simulink model "pfc_desktop_hdl"  (R2024b)
settings: Solver=FixedStepDiscrete  StartTime=0.0  StopTime=.4  RelTol=1e-3
InitFcn:
  | fidelity_pfc_vals;
values from neighbouring files (symbols this model uses):
  fsw = 65    [fidelity_pfc_vals.m]
  Gs = 2e-2    (= 0.02)    [fidelity_pfc_vals.m]
  s = 1    [fidelity_pfc_vals.m]
  t_ss = tsw/30    (= 5.12820512821e-07)    [fidelity_pfc_vals.m]
  tsw = 1/(fsw*1e3)    (= 1.53846153846e-05)    [fidelity_pfc_vals.m]
undefined symbols (not defined in the file or in its folder): a, b, c, DiscIntNeverNeededParam
libraries: fl_lib x37, nesl_utility x31, hdlsllib x6, mcbcontrolslib x5, ee_lib x5, dspsrcs4 x3, slpidlib x2, simulink x1, spsSVPWMGenerator2LevelLib x1, spsPLL3phLib x1
(part 1 of 2)
settings Model: Creator=angro  LastModifiedBy=Angel
settings OptimizationCC: BlockReduction=off  ConditionallyExecuteInputs=off  DefaultParameterBehavior=Inlined
settings DebuggingCC: AlgebraicLoopMsg=error
settings HardwareCC: ProdBitPerPointer=32  ProdBitPerSizeT=32  ProdBitPerPtrDiffT=32  ProdLargestAtomicFloat=None  ProdIntDivRoundTo=Undefined  ProdEndianess=Unspecified  ProdWordSize=32  ProdHWDeviceType=ASIC/FPGA->ASIC/FPGA  TargetBitPerPointer=64  TargetBitPerSizeT=64  TargetBitPerPtrDiffT=64  TargetLongLongMode=on  TargetIntDivRoundTo=Zero  TargetEndianess=LittleEndian  TargetWordSize=64  TargetHWDeviceType=Custom Processor->MATLAB Host Computer  ProdEqTarget=off

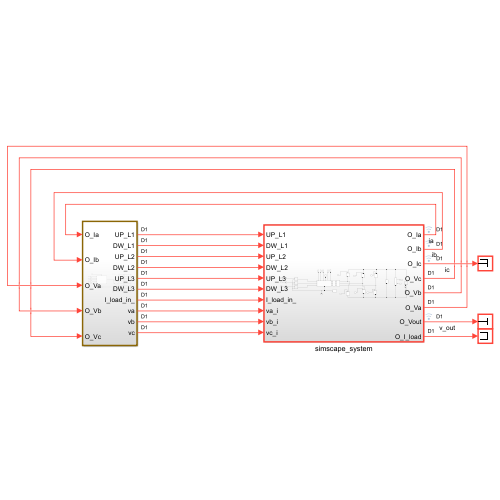
[thumbnail: Simulink's stored preview of the top-level diagram]
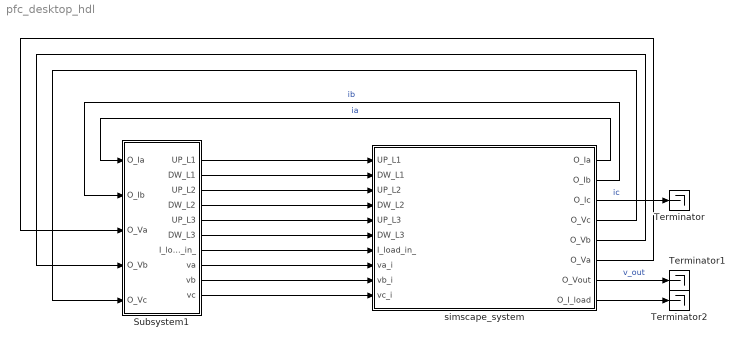
== system pfc_desktop_hdl ==
  Subsystem1 : Subsystem
  Terminator : Terminator
  Terminator1 : Terminator
  Terminator2 : Terminator
  simscape_system : Subsystem
  wires:
  simscape_system/1(O_Ia) -> Subsystem1/1(O_Ia)  "ia"
  simscape_system/6(O_Va) -> Subsystem1/3(O_Va)
  Subsystem1/5(UP_L3) -> simscape_system/5(UP_L3)
  Subsystem1/10(vc) -> simscape_system/10(vc_i)
  simscape_system/2(O_Ib) -> Subsystem1/2(O_Ib)  "ib"
  Subsystem1/9(vb) -> simscape_system/9(vb_i)
  Subsystem1/7(I_load_in_) -> simscape_system/7(I_load_in_)
  Subsystem1/3(UP_L2) -> simscape_system/3(UP_L2)
  Subsystem1/4(DW_L2) -> simscape_system/4(DW_L2)
  simscape_system/4(O_Vc) -> Subsystem1/5(O_Vc)
  Subsystem1/2(DW_L1) -> simscape_system/2(DW_L1)
  simscape_system/5(O_Vb) -> Subsystem1/4(O_Vb)
  simscape_system/3(O_Ic) -> Terminator/1  "ic"
  Subsystem1/6(DW_L3) -> simscape_system/6(DW_L3)
  simscape_system/8(O_I_load) -> Terminator2/1
  Subsystem1/1(UP_L1) -> simscape_system/1(UP_L1)
  simscape_system/7(O_Vout) -> Terminator1/1  "v_out"
  Subsystem1/8(va) -> simscape_system/8(va_i)

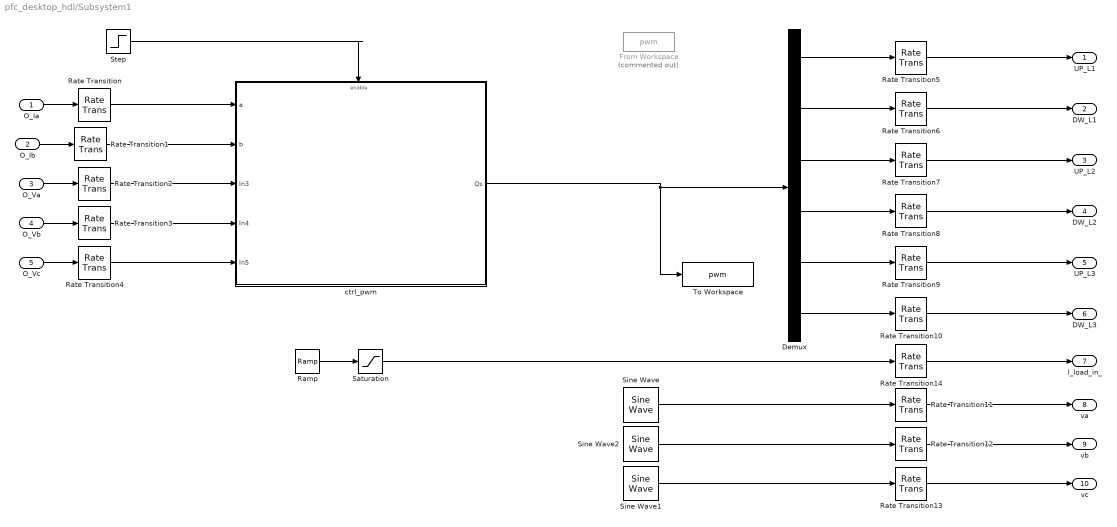
== system pfc_desktop_hdl/Subsystem1 ==
  O_Ia : Inport
  O_Ib : Inport  Port=2
  O_Va : Inport  Port=3
  O_Vb : Inport  Port=4
  O_Vc : Inport  Port=5
  Demux : Demux  Outputs=6
  From Workspace : FromWorkspace  Commented=on  VariableName=pwm  SampleTime=t_ss  Interpolate=off  ZeroCross=off  OutputAfterFinalValue=Holding final value
  Ramp : simulink/Sources/Ramp  slope=1/50  start=2/50  InitialOutput=0
  Rate Transition{,1..4,14} (6 alike) : RateTransition  OutPortSampleTime=t_ss
  Rate Transition{5..13} (9 alike) : RateTransition
  Saturation : Saturate  UpperLimit=2
  Sine Wave : dspsrcs4/Sine Wave  Amplitude=325  Frequency=50  Phase=0  SampleMode=Discrete  OutComplex=Real  CompMethod=Table lookup  TableSize=Speed  SampleTime=tsw  SamplesPerFrame=1  ResetState=Restart at time zero  OutputFrames=off  dataType=double  wordLen=16  udDataType=sfix(16)  fracBitsMode=Best precision  numFracBits=15  OutDataTypeStr=double  LastOutDataTypeStr=double
  Sine Wave1 : dspsrcs4/Sine Wave  Amplitude=325  Frequency=50  Phase=2*pi/3  SampleMode=Discrete  OutComplex=Real  CompMethod=Table lookup  TableSize=Speed  SampleTime=tsw  SamplesPerFrame=1  ResetState=Restart at time zero  OutputFrames=off  dataType=double  wordLen=16  udDataType=sfix(16)  fracBitsMode=Best precision  numFracBits=15  OutDataTypeStr=double  LastOutDataTypeStr=double
  Sine Wave2 : dspsrcs4/Sine Wave  Amplitude=325  Frequency=50  Phase=-2*pi/3  SampleMode=Discrete  OutComplex=Real  CompMethod=Table lookup  TableSize=Speed  SampleTime=tsw  SamplesPerFrame=1  ResetState=Restart at time zero  OutputFrames=off  dataType=double  wordLen=16  udDataType=sfix(16)  fracBitsMode=Best precision  numFracBits=15  OutDataTypeStr=double  LastOutDataTypeStr=double
  Step : Step  Time=2/50  SampleTime=0
  To Workspace : ToWorkspace  VariableName=pwm  SaveFormat=Timeseries  SampleTime=-1
  ctrl_pwm : Subsystem
  UP_L1 : Outport
  DW_L1 : Outport  Port=2
  UP_L2 : Outport  Port=3
  DW_L2 : Outport  Port=4
  UP_L3 : Outport  Port=5
  DW_L3 : Outport  Port=6
  I_load_in_ : Outport  Port=7
  va : Outport  Port=8
  vb : Outport  Port=9
  vc : Outport  Port=10
  wires:
  Demux/5 -> Rate Transition9/1
  Demux/1 -> Rate Transition5/1
  Demux/6 -> Rate Transition10/1
  Demux/4 -> Rate Transition8/1
  Demux/3 -> Rate Transition7/1
  Demux/2 -> Rate Transition6/1
  O_Ia/1 -> Rate Transition/1
  O_Ib/1 -> Rate Transition1/1
  O_Va/1 -> Rate Transition2/1
  O_Vb/1 -> Rate Transition3/1
  O_Vc/1 -> Rate Transition4/1
  Rate Transition5/1 -> UP_L1/1
  Rate Transition6/1 -> DW_L1/1
  Rate Transition7/1 -> UP_L2/1
  Rate Transition8/1 -> DW_L2/1
  Rate Transition9/1 -> UP_L3/1
  Rate Transition10/1 -> DW_L3/1
  Saturation/1 -> Rate Transition14/1
  Sine Wave/1 -> Rate Transition11/1
  Sine Wave2/1 -> Rate Transition12/1
  Sine Wave1/1 -> Rate Transition13/1
  Rate Transition11/1 -> va/1
  Rate Transition12/1 -> vb/1
  Rate Transition13/1 -> vc/1
  ctrl_pwm/1(Qs) -> Demux/1, To Workspace/1
  Rate Transition/1 -> ctrl_pwm/1(a)
  Rate Transition1/1 -> ctrl_pwm/2(b)
  Rate Transition2/1 -> ctrl_pwm/3(In3)
  Rate Transition3/1 -> ctrl_pwm/4(In4)
  Rate Transition4/1 -> ctrl_pwm/5(In5)
  Step/1 -> ctrl_pwm/Enable
  Rate Transition14/1 -> I_load_in_/1
  Ramp/1 -> Saturation/1

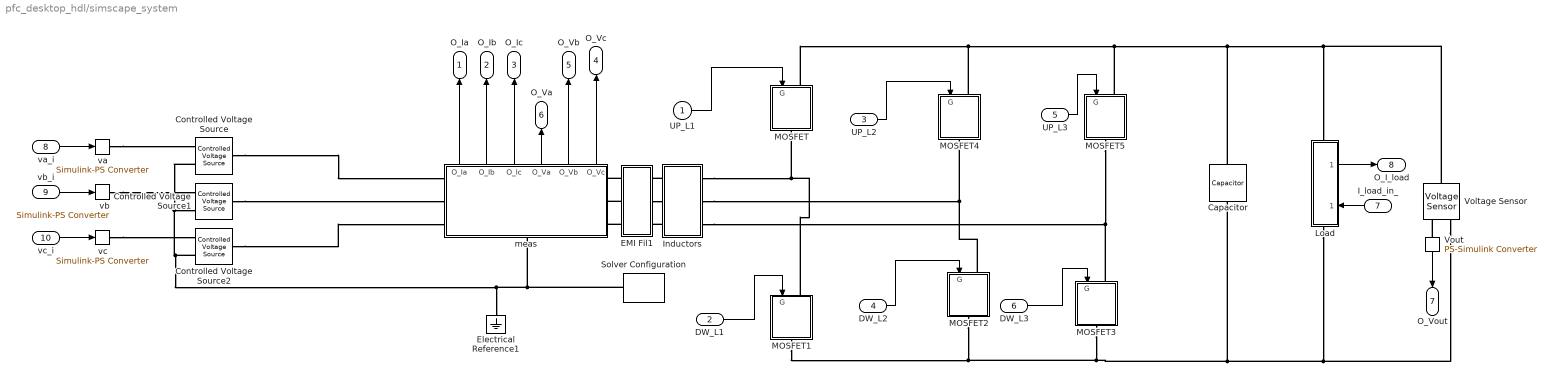
== system pfc_desktop_hdl/simscape_system ==
  UP_L1 : Inport
  DW_L1 : Inport  Port=2
  UP_L2 : Inport  Port=3
  DW_L2 : Inport  Port=4
  UP_L3 : Inport  Port=5
  DW_L3 : Inport  Port=6
  I_load_in_ : Inport  Port=7
  va_i : Inport  Port=8
  vb_i : Inport  Port=9
  vc_i : Inport  Port=10
  Capacitor : ee_lib/Passive/Capacitor  cap_option=ee.enum.passive.capacitor.capOption.const  c=c_out uF  Cvec=[1e-05, 1e-06] F  Vvec=[0, 10] V  CV_table_symmetry=1  f_vec=[1, 10] kHz  DFext_vec=[.8, 1.2]  enable_C_tol=0  averaging_period=0 s  C_tol=5  tol_distribution=1  nSigma=4  r=1e-3*6 Ohm  g=0 1/Ohm  enable_operating_limits=0  operating_limit_action=2  max_working_voltage_range=[-25, 25] V  power_rating=1 W  maxTemperature=85 degC  thermalEnable=false  thermalMass=1 J/K  fault_action=simscape.enum.assert.action.none  t_fault=1 s  i_specify=off  i_priority=None  i=0 A  i_nominal_specify=off  i_nominal_value=1  i_nominal_unit=A  v_specify=off  v_priority=None  v=0 V  v_nominal_specify=off  v_nominal_value=1  v_nominal_unit=V  vc_specify=on  vc_priority=High  vc=580 V  vc_nominal_specify=off  vc_nominal_value=1  vc_nominal_unit=V  T_specify=off  T_priority=None  T=298.15 K  T_nominal_specify=off  T_nominal_value=1  T_nominal_unit=K
  Controlled Voltage Source : fl_lib/Electrical/Electrical Sources/Controlled Voltage Source
  Controlled Voltage Source1 : fl_lib/Electrical/Electrical Sources/Controlled Voltage Source
  Controlled Voltage Source2 : fl_lib/Electrical/Electrical Sources/Controlled Voltage Source
  EMI Fil1 : Subsystem
  Electrical Reference1 : fl_lib/Electrical/Electrical Elements/Electrical Reference
  Inductors : Subsystem
  Load : Subsystem
      settings: PortSchema="{\"entries\":[{\"content\":{\"sides\":[{\"content\":{\"connectorIds\":[\"LConn1\"]},\"type\":\"ConnectorPlacement.EquallySpacedRectSide\",\"uuid\":\"effb2338-687f-46f5-a36d-064d1cdd1f89\"},{\"content\":{\"connectorIds\":[\"RConn1\"],\"side\":\"RIGHT\"},\"type\":\"ConnectorPlacement.EquallySpacedRectSide\",\"uuid\":\"901d8297-0f3f-4280-ade7-978b42e696ee\"},{\"content\":{\"side\":\"TOP\"},\"type\":\"ConnectorPlacement.EquallySpacedRectSide\",\"uuid\":\"94ece1e5-b3d1-4ff8-a800-be801e6d950f\"},{\"content\":{\"connectorIds\":[\"In1\",\"Out1\"],\"side\":\"BOTTOM\"},\"type\":\"ConnectorPlacement.EquallySpacedRectSide\",\"uuid\":\"36082d89-7906-4f78-be00-891e05fea0eb\"}]},\"type\":\"ConnectorPlacement.EquallySpacedConnector\",\"uuid\":\"9e7f386b-2a06-43cf-bdf5-65e67bd802eb\"}],\"packageUris\":[\"http://schema.mathworks.com/mf0/Connector/R2020b\"],\"version\":\"1.0\"}"
  MOSFET : Subsystem
      settings: CopyFcn=set_param(gcb, 'LinkStatus', 'none');
  MOSFET1 : Subsystem
      settings: CopyFcn=set_param(gcb, 'LinkStatus', 'none');
  MOSFET2 : Subsystem
      settings: CopyFcn=set_param(gcb, 'LinkStatus', 'none');
  MOSFET3 : Subsystem
      settings: CopyFcn=set_param(gcb, 'LinkStatus', 'none');
  MOSFET4 : Subsystem
      settings: CopyFcn=set_param(gcb, 'LinkStatus', 'none');
  MOSFET5 : Subsystem
      settings: CopyFcn=set_param(gcb, 'LinkStatus', 'none');
  Solver Configuration : nesl_utility/Solver Configuration  PhysicalDomain=network_engine_domain  SubClassName=solver  LeftPortType=input  RightPortType=generic  Tones=[]  Harmonics=[]  SimulateNoise=off  Profile=off  UseLocalSampling=off  EnableSwitchedLinearOptims=on  FrequencyDomain=off  UseCCode=off  RelTol=0.001  AbsTol=1e-06  MinStep=1e-09  ToWorkspace=off  RevertToSquareIcSolve=off  NumHomotopyIterations=100  PhasorMode=off  PhasorModeNumHarmonics=1  ConsistencySolver=NEWTON_FTOL  IndexReductionMethod=None  DoDC=off  ResidualTolerance=1e-6  ConsistencyTolSource=GLOBAL  ConsistencyAbsTol=0.001  ConsistencyRelTol=0.001  ConsistencyTolFactor=0.001  UseLocalSolver=on  LocalSolverChoice=NE_BACKWARD_EULER_ADVANCER  ResolveIndetEquations=on  FunctionEvalNumThread=1  LocalSolverSampleTime=t_ss  DoFixedCost=on  MaxNonlinIter=1  MaxModeIter=10  ComputeImpulses=off  ImpulseIterations=2  LinearAlgebra=auto  LinearAlgebraNumThread=0  EquationFormulation=NE_TIME_EF  DelaysMemoryBudget=1024  AutomaticFiltering=off  FilteringTimeConstant=0.001  PartitionStorageMethod=EXHAUSTIVE  PartitionMemoryBudget=1024  PartitionMethod=ROBUST  MultibodyUseLocalSolver=off  MultibodyLocalSolverChoice=ODE1  MultibodyLocalSolverSampleTime=0.001
  Voltage Sensor : fl_lib/Electrical/Electrical Sensors/Voltage Sensor
  Vout : nesl_utility/PS-Simulink Converter  PhysicalDomain=network_engine_domain  SubClassName=ps_output  LeftPortType=input  RightPortType=output  PseudoPeriodic=off  Frequencies=[]  VectorFormat=1-D array  Unit=V  AffineConversion=off
  meas : Subsystem
      settings: PortSchema="{\"entries\":[{\"content\":{\"sides\":[{\"content\":{\"connectorIds\":[\"LConn1\",\"LConn2\",\"LConn3\"]},\"type\":\"ConnectorPlacement.EquallySpacedRectSide\",\"uuid\":\"63fb0446-2195-41ce-9f27-949cb83cb3c9\"},{\"content\":{\"connectorIds\":[\"RConn1\",\"RConn2\",\"RConn3\"],\"side\":\"RIGHT\"},\"type\":\"ConnectorPlacement.EquallySpacedRectSide\",\"uuid\":\"9968c418-1dbf-4d06-ba5c-e609e6b84d90\"},{\"content\":{\"connectorIds\":[\"Out1\",\"Out2\",\"Out3\",\"Out4\",\"Out5\",\"Out6\"],\"side\":\"TOP\"},\"type\":\"ConnectorPlacement.EquallySpacedRectSide\",\"uuid\":\"bf7c2fdb-620d-435f-9b2a-06b2c14c987c\"},{\"content\":{\"connectorIds\":[\"RConn4\"],\"side\":\"BOTTOM\"},\"type\":\"ConnectorPlacement.EquallySpacedRectSide\",\"uuid\":\"eb9cce3f-153e-47a2-a171-a4890e03f4a1\"}]},\"type\":\"ConnectorPlacement.EquallySpacedConnector\",\"uuid\":\"4b9ac32f-b167-4dce-a874-653844c6cf4c\"}],\"packageUris\":[\"http://schema.mathworks.com/mf0/Connector/R2020b\"],\"version\":\"1.0\"}"
  va : nesl_utility/Simulink-PS Converter  PhysicalDomain=network_engine_domain  SubClassName=ps_input  LeftPortType=input  RightPortType=output  PseudoPeriodic=off  Frequencies=[]  NoiseDistribution=none  NoiseParameters=[]  Unit=V  AffineConversion=off  FilteringAndDerivatives=zero  SimscapeFilterOrder=1  InputFilterTimeConstant=0.001  UdotUserProvided=0
  vb : nesl_utility/Simulink-PS Converter  PhysicalDomain=network_engine_domain  SubClassName=ps_input  LeftPortType=input  RightPortType=output  PseudoPeriodic=off  Frequencies=[]  NoiseDistribution=none  NoiseParameters=[]  Unit=V  AffineConversion=off  FilteringAndDerivatives=zero  SimscapeFilterOrder=1  InputFilterTimeConstant=0.001  UdotUserProvided=0
  vc : nesl_utility/Simulink-PS Converter  PhysicalDomain=network_engine_domain  SubClassName=ps_input  LeftPortType=input  RightPortType=output  PseudoPeriodic=off  Frequencies=[]  NoiseDistribution=none  NoiseParameters=[]  Unit=V  AffineConversion=off  FilteringAndDerivatives=zero  SimscapeFilterOrder=1  InputFilterTimeConstant=0.001  UdotUserProvided=0
  O_Ia : Outport
  O_Ib : Outport  Port=2
  O_Ic : Outport  Port=3
  O_Vc : Outport  Port=4
  O_Vb : Outport  Port=5
  O_Va : Outport  Port=6
  O_Vout : Outport  Port=7
  O_I_load : Outport  Port=8
  wires:
  DW_L1/1 -> MOSFET1/1(G)
  UP_L3/1 -> MOSFET5/1(G)
  UP_L2/1 -> MOSFET4/1(G)
  DW_L3/1 -> MOSFET3/1(G)
  UP_L1/1 -> MOSFET/1(G)
  DW_L2/1 -> MOSFET2/1(G)
  Vout/1 -> O_Vout/1
  I_load_in_/1 -> Load/1(I_load_in_)
  meas/1(O_Ia) -> O_Ia/1
  meas/2(O_Ib) -> O_Ib/1
  meas/3(O_Ic) -> O_Ic/1
  meas/6(O_Vc) -> O_Vc/1
  meas/5(O_Vb) -> O_Vb/1
  meas/4(O_Va) -> O_Va/1
  va_i/1 -> va/1
  vb_i/1 -> vb/1
  vc_i/1 -> vc/1
  Load/1(O_I_load) -> O_I_load/1
  connections:
  Controlled Voltage Source/RConn2 -- Electrical Reference1/LConn1 -- Solver Configuration/RConn1 -- meas/RConn4 -- Controlled Voltage Source2/RConn2 -- Controlled Voltage Source1/RConn2
  Inductors/LConn1 -- EMI Fil1/RConn1
  EMI Fil1/RConn2 -- Inductors/LConn2
  Inductors/LConn3 -- EMI Fil1/RConn3
  Capacitor/LConn1 -- MOSFET5/LConn1 -- MOSFET4/LConn1 -- MOSFET/LConn1 -- Voltage Sensor/LConn1 -- Load/RConn1
  va/RConn1 -- Controlled Voltage Source/RConn1
  vb/RConn1 -- Controlled Voltage Source1/RConn1
  vc/RConn1 -- Controlled Voltage Source2/RConn1
  Controlled Voltage Source/LConn1 -- meas/LConn1
  Controlled Voltage Source1/LConn1 -- meas/LConn2
  Controlled Voltage Source2/LConn1 -- meas/LConn3
  EMI Fil1/LConn1 -- meas/RConn1
  EMI Fil1/LConn2 -- meas/RConn2
  EMI Fil1/LConn3 -- meas/RConn3
  Inductors/RConn1 -- MOSFET1/LConn1 -- MOSFET/RConn1
  Inductors/RConn2 -- MOSFET4/RConn1 -- MOSFET2/LConn1
  Inductors/RConn3 -- MOSFET5/RConn1 -- MOSFET3/LConn1
  Load/LConn1 -- Voltage Sensor/RConn2 -- MOSFET3/RConn1 -- MOSFET2/RConn1 -- MOSFET1/RConn1 -- Capacitor/RConn1
  Vout/LConn1 -- Voltage Sensor/RConn1

== system pfc_desktop_hdl/Subsystem1/ctrl_pwm ==
  a : Inport
  b : Inport  Port=2
  In3 : Inport  Port=3
  In4 : Inport  Port=4
  In5 : Inport  Port=5
  Enable : EnablePort
  PI_CTRL : Subsystem
  SVPWM : Subsystem
  transforms : Subsystem
  Qs : Outport
  wires:
  transforms/1(id) -> PI_CTRL/1(id)
  transforms/3(angle) -> SVPWM/2(angle)
  PI_CTRL/1(Vd_inductor) -> SVPWM/1(Vd_inductor)
  a/1 -> transforms/1(a)
  In5/1 -> transforms/5(In5)
  transforms/2(iq) -> PI_CTRL/2(iq)
  SVPWM/1(P) -> Qs/1  "Qs"
  PI_CTRL/2(Vq_inductor) -> SVPWM/3(Vq_inductor)
  b/1 -> transforms/2(b)
  In3/1 -> transforms/3(In3)
  In4/1 -> transforms/4(In4)

== system pfc_desktop_hdl/simscape_system/EMI Fil1 ==
  Coupled Lines (Three-Phase) : ee_lib/Passive/Lines/Coupled Lines (Three-Phase)  prm=1  La=1e-3 H  Lb=1e-3 H  Lc=1e-3 H  L=10 mH  Lmab=3e-4 H  Lmac=3e-4 H  Lmbc=3e-4 H  Lm=0 mH  Ra=0.001 Ohm  Rb=0.001 Ohm  Rc=0.001 Ohm  R=0.001 Ohm  Rm=0 Ohm  Ga=1e-9 1/Ohm  Gb=1e-9 1/Ohm  Gc=1e-9 1/Ohm  G=1e-9 1/Ohm  I_L_specify=off  I_L_priority=High  I_L=[0, 0, 0] A  I_L_nominal_specify=off  I_L_nominal_value=1  I_L_nominal_unit=A  i_La_specify=off  i_La_priority=High  i_La=0 A  i_La_nominal_specify=off  i_La_nominal_value=1  i_La_nominal_unit=A  i_Lb_specify=off  i_Lb_priority=High  i_Lb=0 A  i_Lb_nominal_specify=off  i_Lb_nominal_value=1  i_Lb_nominal_unit=A  i_Lc_specify=off  i_Lc_priority=High  i_Lc=0 A  i_Lc_nominal_specify=off  i_Lc_nominal_value=1  i_Lc_nominal_unit=A
      settings: InternalSimscapePortConfiguration="{\"Bottom\":[],\"Left\":[{\"id\":\"a1\",\"label\":\"a1\",\"type\":\"foundation.electrical.electrical\"},{\"id\":\"b1\",\"label\":\"b1\",\"type\":\"foundation.electrical.electrical\"},{\"id\":\"c1\",\"label\":\"c1\",\"type\":\"foundation.electrical.electrical\"}],\"Right\":[{\"id\":\"a2\",\"label\":\"a2\",\"type\":\"foundation.electrical.electrical\"},{\"id\":\"b2\",\"label\":\"b2\",\"type\":\"foundation.electrical.electrical\"},{\"id\":\"c2\",\"label\":\"c2\",\"type\":\"foundation.electrical.electrical\"}],\"Top\":[]}"
  +A : PMIOPort  Side=Left
  +B : PMIOPort  Port=2  Side=Left
  +C : PMIOPort  Port=3  Side=Left
  -A : PMIOPort  Port=4  Side=Right
  -B : PMIOPort  Port=5  Side=Right
  -C : PMIOPort  Port=6  Side=Right
  connections:
  Coupled Lines (Three-Phase)/LConn1 -- +A/RConn1
  +C/RConn1 -- Coupled Lines (Three-Phase)/LConn3
  -C/RConn1 -- Coupled Lines (Three-Phase)/RConn3
  -B/RConn1 -- Coupled Lines (Three-Phase)/RConn2
  +B/RConn1 -- Coupled Lines (Three-Phase)/LConn2
  -A/RConn1 -- Coupled Lines (Three-Phase)/RConn1

== system pfc_desktop_hdl/simscape_system/Inductors ==
  Inductor : ee_lib/Passive/Inductor  l=l_ind uH  enable_L_tol=0  L_tol=0  tol_distribution=1  nSigma=4  r=1e-3 Ohm  g=1e-9 1/Ohm  enable_operating_limits=0  operating_limit_action=2  max_working_current=1 A  power_rating=1 W  fault_action=simscape.enum.assert.action.none  t_fault=1 s  i_L_specify=off  i_L_priority=High  i_L=0 A  i_L_nominal_specify=off  i_L_nominal_value=1  i_L_nominal_unit=A
  Inductor1 : ee_lib/Passive/Inductor  l=l_ind uH  enable_L_tol=0  L_tol=0  tol_distribution=1  nSigma=4  r=1e-3 Ohm  g=1e-9 1/Ohm  enable_operating_limits=0  operating_limit_action=2  max_working_current=1 A  power_rating=1 W  fault_action=simscape.enum.assert.action.none  t_fault=1 s  i_L_specify=off  i_L_priority=High  i_L=0 A  i_L_nominal_specify=off  i_L_nominal_value=1  i_L_nominal_unit=A
  Inductor2 : ee_lib/Passive/Inductor  l=l_ind uH  enable_L_tol=0  L_tol=0  tol_distribution=1  nSigma=4  r=1e-3 Ohm  g=1e-9 1/Ohm  enable_operating_limits=0  operating_limit_action=2  max_working_current=1 A  power_rating=1 W  fault_action=simscape.enum.assert.action.none  t_fault=1 s  i_L_specify=off  i_L_priority=High  i_L=0 A  i_L_nominal_specify=off  i_L_nominal_value=1  i_L_nominal_unit=A
  IAout : PMIOPort  Side=Right
  IA : PMIOPort  Port=2  Side=Left
  Ib : PMIOPort  Port=3  Side=Left
  IBout : PMIOPort  Port=4  Side=Right
  IC : PMIOPort  Port=5  Side=Left
  ICout : PMIOPort  Port=6  Side=Right
  connections:
  Ib/RConn1 -- Inductor/LConn1
  IBout/RConn1 -- Inductor/RConn1
  IAout/RConn1 -- Inductor2/RConn1
  Inductor2/LConn1 -- IA/RConn1
  Inductor1/LConn1 -- IC/RConn1
  ICout/RConn1 -- Inductor1/RConn1

== system pfc_desktop_hdl/simscape_system/Load ==
  I_load_in_ : Inport
  Controlled Current Source : fl_lib/Electrical/Electrical Sources/Controlled Current Source
  Current Sensor : fl_lib/Electrical/Electrical Sensors/Current Sensor
  I_load : nesl_utility/PS-Simulink Converter  PhysicalDomain=network_engine_domain  SubClassName=ps_output  LeftPortType=input  RightPortType=output  PseudoPeriodic=off  Frequencies=[]  VectorFormat=1-D array  Unit=inherit  AffineConversion=off
  I_load_in : nesl_utility/Simulink-PS Converter  PhysicalDomain=network_engine_domain  SubClassName=ps_input  LeftPortType=input  RightPortType=output  PseudoPeriodic=off  Frequencies=[]  NoiseDistribution=none  NoiseParameters=[]  Unit=1  AffineConversion=off  FilteringAndDerivatives=zero  SimscapeFilterOrder=1  InputFilterTimeConstant=0.001  UdotUserProvided=0
  Iout : PMIOPort  Side=Left
  Iin : PMIOPort  Port=2  Side=Right
  O_I_load : Outport
  wires:
  I_load_in_/1 -> I_load_in/1
  I_load/1 -> O_I_load/1
  connections:
  Current Sensor/LConn1 -- Controlled Current Source/LConn1
  Controlled Current Source/RConn2 -- Iin/RConn1
  I_load_in/RConn1 -- Controlled Current Source/RConn1
  I_load/LConn1 -- Current Sensor/RConn1
  Current Sensor/RConn2 -- Iout/RConn1

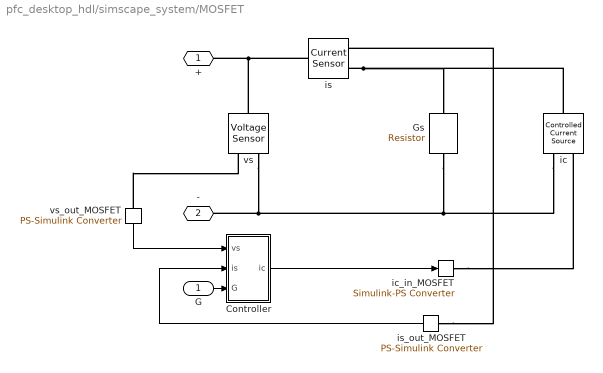
== system pfc_desktop_hdl/simscape_system/MOSFET ==
  G : Inport
  Controller : Subsystem
  Gs : fl_lib/Electrical/Electrical Elements/Resistor  R=1/Gs Ohm  i_specify=off  i_priority=None  i=0 A  i_nominal_specify=off  i_nominal_value=1  i_nominal_unit=A  v_specify=off  v_priority=None  v=0 V  v_nominal_specify=off  v_nominal_value=1  v_nominal_unit=V
  ic : fl_lib/Electrical/Electrical Sources/Controlled Current Source
  ic_in_MOSFET : nesl_utility/Simulink-PS Converter  PhysicalDomain=network_engine_domain  SubClassName=ps_input  LeftPortType=input  RightPortType=output  PseudoPeriodic=off  Frequencies=[]  NoiseDistribution=none  NoiseParameters=[]  Unit=A  AffineConversion=off  FilteringAndDerivatives=provide  SimscapeFilterOrder=1  InputFilterTimeConstant=0.001  UdotUserProvided=0
  is : fl_lib/Electrical/Electrical Sensors/Current Sensor
  is_out_MOSFET : nesl_utility/PS-Simulink Converter  PhysicalDomain=network_engine_domain  SubClassName=ps_output  LeftPortType=input  RightPortType=output  PseudoPeriodic=off  Frequencies=[]  VectorFormat=1-D array  Unit=A  AffineConversion=off
  vs : fl_lib/Electrical/Electrical Sensors/Voltage Sensor
  vs_out_MOSFET : nesl_utility/PS-Simulink Converter  PhysicalDomain=network_engine_domain  SubClassName=ps_output  LeftPortType=input  RightPortType=output  PseudoPeriodic=off  Frequencies=[]  VectorFormat=1-D array  Unit=V  AffineConversion=off
  + : PMIOPort  Side=Left
  - : PMIOPort  Port=2  Side=Right
  wires:
  Controller/1(ic) -> ic_in_MOSFET/1
  G/1 -> Controller/3(G)
  is_out_MOSFET/1 -> Controller/2(is)
  vs_out_MOSFET/1 -> Controller/1(vs)
  connections:
  is_out_MOSFET/LConn1 -- is/RConn1
  vs_out_MOSFET/LConn1 -- vs/RConn1
  ic_in_MOSFET/RConn1 -- ic/RConn1
  is/LConn1 -- +/RConn1 -- vs/LConn1
  ic/RConn2 -- Gs/RConn1 -- -/RConn1 -- vs/RConn2
  is/RConn2 -- Gs/LConn1 -- ic/LConn1

== system pfc_desktop_hdl/simscape_system/MOSFET1 ==
  G : Inport
  Controller : Subsystem
  Gs : fl_lib/Electrical/Electrical Elements/Resistor  R=1/Gs Ohm  i_specify=off  i_priority=None  i=0 A  i_nominal_specify=off  i_nominal_value=1  i_nominal_unit=A  v_specify=off  v_priority=None  v=0 V  v_nominal_specify=off  v_nominal_value=1  v_nominal_unit=V
  ic : fl_lib/Electrical/Electrical Sources/Controlled Current Source
  ic_in_MOSFET : nesl_utility/Simulink-PS Converter  PhysicalDomain=network_engine_domain  SubClassName=ps_input  LeftPortType=input  RightPortType=output  PseudoPeriodic=off  Frequencies=[]  NoiseDistribution=none  NoiseParameters=[]  Unit=A  AffineConversion=off  FilteringAndDerivatives=provide  SimscapeFilterOrder=1  InputFilterTimeConstant=0.001  UdotUserProvided=0
  is : fl_lib/Electrical/Electrical Sensors/Current Sensor
  is_out_MOSFET : nesl_utility/PS-Simulink Converter  PhysicalDomain=network_engine_domain  SubClassName=ps_output  LeftPortType=input  RightPortType=output  PseudoPeriodic=off  Frequencies=[]  VectorFormat=1-D array  Unit=A  AffineConversion=off
  vs : fl_lib/Electrical/Electrical Sensors/Voltage Sensor
  vs_out_MOSFET : nesl_utility/PS-Simulink Converter  PhysicalDomain=network_engine_domain  SubClassName=ps_output  LeftPortType=input  RightPortType=output  PseudoPeriodic=off  Frequencies=[]  VectorFormat=1-D array  Unit=V  AffineConversion=off
  + : PMIOPort  Side=Left
  - : PMIOPort  Port=2  Side=Right
  wires:
  vs_out_MOSFET/1 -> Controller/1(vs)
  is_out_MOSFET/1 -> Controller/2(is)
  G/1 -> Controller/3(G)
  Controller/1(ic) -> ic_in_MOSFET/1
  connections:
  ic/LConn1 -- Gs/LConn1 -- is/RConn2
  vs/RConn2 -- -/RConn1 -- Gs/RConn1 -- ic/RConn2
  vs/LConn1 -- +/RConn1 -- is/LConn1
  ic_in_MOSFET/RConn1 -- ic/RConn1
  vs_out_MOSFET/LConn1 -- vs/RConn1
  is_out_MOSFET/LConn1 -- is/RConn1

== system pfc_desktop_hdl/simscape_system/MOSFET2 ==
  G : Inport
  Controller : Subsystem
  Gs : fl_lib/Electrical/Electrical Elements/Resistor  R=1/Gs Ohm  i_specify=off  i_priority=None  i=0 A  i_nominal_specify=off  i_nominal_value=1  i_nominal_unit=A  v_specify=off  v_priority=None  v=0 V  v_nominal_specify=off  v_nominal_value=1  v_nominal_unit=V
  ic : fl_lib/Electrical/Electrical Sources/Controlled Current Source
  ic_in_MOSFET : nesl_utility/Simulink-PS Converter  PhysicalDomain=network_engine_domain  SubClassName=ps_input  LeftPortType=input  RightPortType=output  PseudoPeriodic=off  Frequencies=[]  NoiseDistribution=none  NoiseParameters=[]  Unit=A  AffineConversion=off  FilteringAndDerivatives=provide  SimscapeFilterOrder=1  InputFilterTimeConstant=0.001  UdotUserProvided=0
  is : fl_lib/Electrical/Electrical Sensors/Current Sensor
  is_out_MOSFET : nesl_utility/PS-Simulink Converter  PhysicalDomain=network_engine_domain  SubClassName=ps_output  LeftPortType=input  RightPortType=output  PseudoPeriodic=off  Frequencies=[]  VectorFormat=1-D array  Unit=A  AffineConversion=off
  vs : fl_lib/Electrical/Electrical Sensors/Voltage Sensor
  vs_out_MOSFET : nesl_utility/PS-Simulink Converter  PhysicalDomain=network_engine_domain  SubClassName=ps_output  LeftPortType=input  RightPortType=output  PseudoPeriodic=off  Frequencies=[]  VectorFormat=1-D array  Unit=V  AffineConversion=off
  + : PMIOPort  Side=Left
  - : PMIOPort  Port=2  Side=Right
  wires:
  Controller/1(ic) -> ic_in_MOSFET/1
  G/1 -> Controller/3(G)
  is_out_MOSFET/1 -> Controller/2(is)
  vs_out_MOSFET/1 -> Controller/1(vs)
  connections:
  is_out_MOSFET/LConn1 -- is/RConn1
  vs_out_MOSFET/LConn1 -- vs/RConn1
  ic_in_MOSFET/RConn1 -- ic/RConn1
  is/LConn1 -- +/RConn1 -- vs/LConn1
  ic/RConn2 -- Gs/RConn1 -- -/RConn1 -- vs/RConn2
  is/RConn2 -- Gs/LConn1 -- ic/LConn1

== system pfc_desktop_hdl/simscape_system/MOSFET3 ==
  G : Inport
  Controller : Subsystem
  Gs : fl_lib/Electrical/Electrical Elements/Resistor  R=1/Gs Ohm  i_specify=off  i_priority=None  i=0 A  i_nominal_specify=off  i_nominal_value=1  i_nominal_unit=A  v_specify=off  v_priority=None  v=0 V  v_nominal_specify=off  v_nominal_value=1  v_nominal_unit=V
  ic : fl_lib/Electrical/Electrical Sources/Controlled Current Source
  ic_in_MOSFET : nesl_utility/Simulink-PS Converter  PhysicalDomain=network_engine_domain  SubClassName=ps_input  LeftPortType=input  RightPortType=output  PseudoPeriodic=off  Frequencies=[]  NoiseDistribution=none  NoiseParameters=[]  Unit=A  AffineConversion=off  FilteringAndDerivatives=provide  SimscapeFilterOrder=1  InputFilterTimeConstant=0.001  UdotUserProvided=0
  is : fl_lib/Electrical/Electrical Sensors/Current Sensor
  is_out_MOSFET : nesl_utility/PS-Simulink Converter  PhysicalDomain=network_engine_domain  SubClassName=ps_output  LeftPortType=input  RightPortType=output  PseudoPeriodic=off  Frequencies=[]  VectorFormat=1-D array  Unit=A  AffineConversion=off
  vs : fl_lib/Electrical/Electrical Sensors/Voltage Sensor
  vs_out_MOSFET : nesl_utility/PS-Simulink Converter  PhysicalDomain=network_engine_domain  SubClassName=ps_output  LeftPortType=input  RightPortType=output  PseudoPeriodic=off  Frequencies=[]  VectorFormat=1-D array  Unit=V  AffineConversion=off
  + : PMIOPort  Side=Left
  - : PMIOPort  Port=2  Side=Right
  wires:
  vs_out_MOSFET/1 -> Controller/1(vs)
  is_out_MOSFET/1 -> Controller/2(is)
  G/1 -> Controller/3(G)
  Controller/1(ic) -> ic_in_MOSFET/1
  connections:
  ic/LConn1 -- Gs/LConn1 -- is/RConn2
  vs/RConn2 -- -/RConn1 -- Gs/RConn1 -- ic/RConn2
  vs/LConn1 -- +/RConn1 -- is/LConn1
  ic_in_MOSFET/RConn1 -- ic/RConn1
  vs_out_MOSFET/LConn1 -- vs/RConn1
  is_out_MOSFET/LConn1 -- is/RConn1

== system pfc_desktop_hdl/simscape_system/MOSFET4 ==
  G : Inport
  Controller : Subsystem
  Gs : fl_lib/Electrical/Electrical Elements/Resistor  R=1/Gs Ohm  i_specify=off  i_priority=None  i=0 A  i_nominal_specify=off  i_nominal_value=1  i_nominal_unit=A  v_specify=off  v_priority=None  v=0 V  v_nominal_specify=off  v_nominal_value=1  v_nominal_unit=V
  ic : fl_lib/Electrical/Electrical Sources/Controlled Current Source
  ic_in_MOSFET : nesl_utility/Simulink-PS Converter  PhysicalDomain=network_engine_domain  SubClassName=ps_input  LeftPortType=input  RightPortType=output  PseudoPeriodic=off  Frequencies=[]  NoiseDistribution=none  NoiseParameters=[]  Unit=A  AffineConversion=off  FilteringAndDerivatives=provide  SimscapeFilterOrder=1  InputFilterTimeConstant=0.001  UdotUserProvided=0
  is : fl_lib/Electrical/Electrical Sensors/Current Sensor
  is_out_MOSFET : nesl_utility/PS-Simulink Converter  PhysicalDomain=network_engine_domain  SubClassName=ps_output  LeftPortType=input  RightPortType=output  PseudoPeriodic=off  Frequencies=[]  VectorFormat=1-D array  Unit=A  AffineConversion=off
  vs : fl_lib/Electrical/Electrical Sensors/Voltage Sensor
  vs_out_MOSFET : nesl_utility/PS-Simulink Converter  PhysicalDomain=network_engine_domain  SubClassName=ps_output  LeftPortType=input  RightPortType=output  PseudoPeriodic=off  Frequencies=[]  VectorFormat=1-D array  Unit=V  AffineConversion=off
  + : PMIOPort  Side=Left
  - : PMIOPort  Port=2  Side=Right
  wires:
  vs_out_MOSFET/1 -> Controller/1(vs)
  is_out_MOSFET/1 -> Controller/2(is)
  G/1 -> Controller/3(G)
  Controller/1(ic) -> ic_in_MOSFET/1
  connections:
  ic/LConn1 -- Gs/LConn1 -- is/RConn2
  vs/RConn2 -- -/RConn1 -- Gs/RConn1 -- ic/RConn2
  vs/LConn1 -- +/RConn1 -- is/LConn1
  ic_in_MOSFET/RConn1 -- ic/RConn1
  vs_out_MOSFET/LConn1 -- vs/RConn1
  is_out_MOSFET/LConn1 -- is/RConn1

== system pfc_desktop_hdl/simscape_system/MOSFET5 ==
  G : Inport
  Controller : Subsystem
  Gs : fl_lib/Electrical/Electrical Elements/Resistor  R=1/Gs Ohm  i_specify=off  i_priority=None  i=0 A  i_nominal_specify=off  i_nominal_value=1  i_nominal_unit=A  v_specify=off  v_priority=None  v=0 V  v_nominal_specify=off  v_nominal_value=1  v_nominal_unit=V
  ic : fl_lib/Electrical/Electrical Sources/Controlled Current Source
  ic_in_MOSFET : nesl_utility/Simulink-PS Converter  PhysicalDomain=network_engine_domain  SubClassName=ps_input  LeftPortType=input  RightPortType=output  PseudoPeriodic=off  Frequencies=[]  NoiseDistribution=none  NoiseParameters=[]  Unit=A  AffineConversion=off  FilteringAndDerivatives=provide  SimscapeFilterOrder=1  InputFilterTimeConstant=0.001  UdotUserProvided=0
  is : fl_lib/Electrical/Electrical Sensors/Current Sensor
  is_out_MOSFET : nesl_utility/PS-Simulink Converter  PhysicalDomain=network_engine_domain  SubClassName=ps_output  LeftPortType=input  RightPortType=output  PseudoPeriodic=off  Frequencies=[]  VectorFormat=1-D array  Unit=A  AffineConversion=off
  vs : fl_lib/Electrical/Electrical Sensors/Voltage Sensor
  vs_out_MOSFET : nesl_utility/PS-Simulink Converter  PhysicalDomain=network_engine_domain  SubClassName=ps_output  LeftPortType=input  RightPortType=output  PseudoPeriodic=off  Frequencies=[]  VectorFormat=1-D array  Unit=V  AffineConversion=off
  + : PMIOPort  Side=Left
  - : PMIOPort  Port=2  Side=Right
  wires:
  Controller/1(ic) -> ic_in_MOSFET/1
  G/1 -> Controller/3(G)
  is_out_MOSFET/1 -> Controller/2(is)
  vs_out_MOSFET/1 -> Controller/1(vs)
  connections:
  is_out_MOSFET/LConn1 -- is/RConn1
  vs_out_MOSFET/LConn1 -- vs/RConn1
  ic_in_MOSFET/RConn1 -- ic/RConn1
  is/LConn1 -- +/RConn1 -- vs/LConn1
  ic/RConn2 -- Gs/RConn1 -- -/RConn1 -- vs/RConn2
  is/RConn2 -- Gs/LConn1 -- ic/LConn1

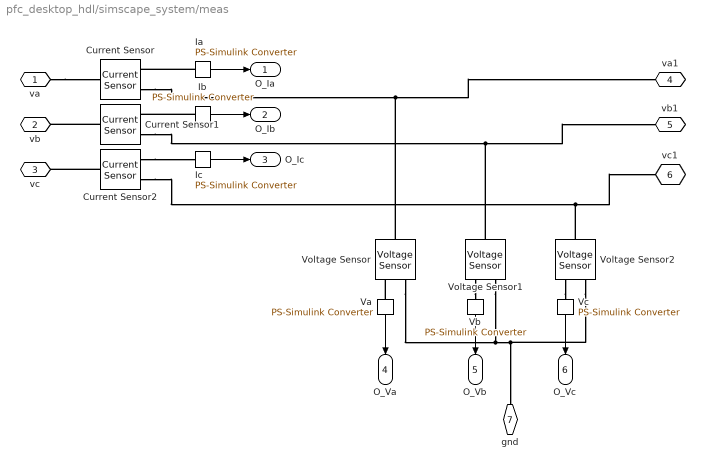
== system pfc_desktop_hdl/simscape_system/meas ==
  Current Sensor : fl_lib/Electrical/Electrical Sensors/Current Sensor
  Current Sensor1 : fl_lib/Electrical/Electrical Sensors/Current Sensor
  Current Sensor2 : fl_lib/Electrical/Electrical Sensors/Current Sensor
  Ia : nesl_utility/PS-Simulink Converter  PhysicalDomain=network_engine_domain  SubClassName=ps_output  LeftPortType=input  RightPortType=output  PseudoPeriodic=off  Frequencies=[]  VectorFormat=1-D array  Unit=A  AffineConversion=off
  Ib : nesl_utility/PS-Simulink Converter  PhysicalDomain=network_engine_domain  SubClassName=ps_output  LeftPortType=input  RightPortType=output  PseudoPeriodic=off  Frequencies=[]  VectorFormat=1-D array  Unit=A  AffineConversion=off
  Ic : nesl_utility/PS-Simulink Converter  PhysicalDomain=network_engine_domain  SubClassName=ps_output  LeftPortType=input  RightPortType=output  PseudoPeriodic=off  Frequencies=[]  VectorFormat=1-D array  Unit=A  AffineConversion=off
  Va : nesl_utility/PS-Simulink Converter  PhysicalDomain=network_engine_domain  SubClassName=ps_output  LeftPortType=input  RightPortType=output  PseudoPeriodic=off  Frequencies=[]  VectorFormat=inherit  Unit=inherit  AffineConversion=off
  Vb : nesl_utility/PS-Simulink Converter  PhysicalDomain=network_engine_domain  SubClassName=ps_output  LeftPortType=input  RightPortType=output  PseudoPeriodic=off  Frequencies=[]  VectorFormat=inherit  Unit=inherit  AffineConversion=off
  Vc : nesl_utility/PS-Simulink Converter  PhysicalDomain=network_engine_domain  SubClassName=ps_output  LeftPortType=input  RightPortType=output  PseudoPeriodic=off  Frequencies=[]  VectorFormat=inherit  Unit=inherit  AffineConversion=off
  Voltage Sensor : fl_lib/Electrical/Electrical Sensors/Voltage Sensor
  Voltage Sensor1 : fl_lib/Electrical/Electrical Sensors/Voltage Sensor
  Voltage Sensor2 : fl_lib/Electrical/Electrical Sensors/Voltage Sensor
  va : PMIOPort  Side=Left
  vb : PMIOPort  Port=2  Side=Left
  vc : PMIOPort  Port=3  Side=Left
  va1 : PMIOPort  Port=4  Side=Right
  vb1 : PMIOPort  Port=5  Side=Right
  vc1 : PMIOPort  Port=6  Side=Right
  gnd : PMIOPort  Port=7  Side=Right
  O_Ia : Outport
  O_Ib : Outport  Port=2
  O_Ic : Outport  Port=3
  O_Va : Outport  Port=4
  O_Vb : Outport  Port=5
  O_Vc : Outport  Port=6
  wires:
  Ia/1 -> O_Ia/1
  Ib/1 -> O_Ib/1
  Ic/1 -> O_Ic/1
  Va/1 -> O_Va/1
  Vb/1 -> O_Vb/1
  Vc/1 -> O_Vc/1
  connections:
  va/RConn1 -- Current Sensor/LConn1
  Current Sensor1/LConn1 -- vb/RConn1
  Current Sensor2/LConn1 -- vc/RConn1
  Ia/LConn1 -- Current Sensor/RConn1
  Ib/LConn1 -- Current Sensor1/RConn1
  Current Sensor2/RConn1 -- Ic/LConn1
  Current Sensor/RConn2 -- Voltage Sensor/LConn1 -- va1/RConn1
  Current Sensor1/RConn2 -- Voltage Sensor1/LConn1 -- vb1/RConn1
  Current Sensor2/RConn2 -- Voltage Sensor2/LConn1 -- vc1/RConn1
  Va/LConn1 -- Voltage Sensor/RConn1
  Voltage Sensor/RConn2 -- Voltage Sensor2/RConn2 -- gnd/RConn1 -- Voltage Sensor1/RConn2
  Voltage Sensor1/RConn1 -- Vb/LConn1
  Voltage Sensor2/RConn1 -- Vc/LConn1

== system pfc_desktop_hdl/Subsystem1/ctrl_pwm/PI_CTRL ==
  id : Inport
  iq : Inport  Port=2
  Add3 : Sum  Inputs=+-
  Add4 : Sum  Inputs=+-
  Constant : Constant  Value=0  SampleTime=t_ss
  Constant1 : Constant  Value=-4  SampleTime=t_ss
  Vd_ctrl : slpidlib/PID Controller  Controller=PI  Form=Parallel  TimeDomain=Discrete-time  UseExternalTs=off  SampleTime=1/(65e3*10)  IntegratorMethod=Backward Euler  FilterMethod=Forward Euler  ControllerParametersSource=internal  P=-1.8  I=-.15  UseKiTs=off  D=0  UseExternalDerivativeSource=off  N=100  UseFilter=on  TunerSelectOption=Transfer Function Based (PID Tuner App)  InitialConditionSource=internal  InitialConditionForIntegrator=0  InitialConditionForFilter=0  DifferentiatorICPrevScaledInput=0  ExternalReset=none  TrackingMode=off  Kt=1  LimitOutput=off  SatLimitsSource=internal  UpperSaturationLimit=5e2  LowerSaturationLimit=-5e2  LinearizeAsGain=on  AntiWindupMode=clamping  Kb=1  LimitIntegrator=off  UpperIntegratorSaturationLimit=inf  LowerIntegratorSaturationLimit=-inf  POutMin=[]  POutMax=[]  IOutMin=[]  IOutMax=[]  DOutMin=[]  DOutMax=[]  NOutMin=[]  NOutMax=[]  SumOutMin=[]  SumOutMax=[]  SaturationOutMin=[]  SaturationOutMax=[]  PParamMin=[]  PParamMax=[]  IParamMin=[]  IParamMax=[]  DParamMin=[]  DParamMax=[]  NParamMin=[]  NParamMax=[]  KbParamMin=[]  KbParamMax=[]  KtParamMin=[]  KtParamMax=[]  KbOutMin=[]  KbOutMax=[]  KtOutMin=[]  KtOutMax=[]  IntegratorOutMin=[]  IntegratorOutMax=[]  FilterOutMin=[]  FilterOutMax=[]  SumI1OutMin=[]  SumI1OutMax=[]  SumI2OutMin=[]  SumI2OutMax=[]  SumI3OutMin=[]  SumI3OutMax=[]  SumI4OutMin=[]  SumI4OutMax=[]  SumDOutMin=[]  SumDOutMax=[]  DifferentiatorOutMin=[]  DifferentiatorOutMax=[]  FilterDiffOutCoefMin=[]  FilterDiffOutCoefMax=[]  ReciprocalOutMin=[]  ReciprocalOutMax=[]  SumDenOutMin=[]  SumDenOutMax=[]  SumNumOutMin=[]  SumNumOutMax=[]  DivideOutMin=[]  DivideOutMax=[]  UdiffTsProdOutMin=[]  UdiffTsProdOutMax=[]  NTsProdOutMin=[]  NTsProdOutMax=[]  UintegralTsProdOutMin=[]  UintegralTsProdOutMax=[]  UngainTsProdOutMin=[]  UngainTsProdOutMax=[]  ClampingZeroOutDataTypeStr=Inherit: Inherit via back propagation  ClampingZeroOutMin=[]  ClampingZeroOutMax=[]  FilterDenConstantOutDataTypeStr=Inherit: Inherit via back propagation  FilterDenConstantOutMin=[]  FilterDenConstantOutMax=[]  PCopyOutDataTypeStr=Inherit: Inherit via back propagation  PCopyOutMin=[]  PCopyOutMax=[]  NCopyOutDataTypeStr=Inherit: Inherit via back propagation  NCopyOutMin=[]  NCopyOutMax=[]  IntegratorContinuousStateAttributes=''  IntegratorStateMustResolveToSignalObject=off  IntegratorRTWStateStorageClass=Auto  FilterContinuousStateAttributes=''  FilterStateMustResolveToSignalObject=off  FilterRTWStateStorageClass=Auto  ParallelPVariant=InternalParameters  IdealPVariant=Disabled  IVariant=InternalParameters  DVariant=Disabled  IntegratorVariant=Discrete  SatVariant=Disabled  AWVariant=Passthrough  PCopyVariant=Disabled  TRVariant=Disabled  FdbkBlocksVariant=Forward  IdealPFdbkVariant=Disabled  SatFdbkVariant=Disabled  DerivativeFilterVariant=Disabled  NVariant=Disabled  NCopyVariant=Disabled_SignalSpec  FilterICVariant=Disabled  IntegratorICVariant=InternalICs  ExternalResetVariant=Disabled  TRSumVariant=Passthrough  SumFdbkVariant=Disabled  SumVariant=Sum_PI  TsampFilterVariant=InternalTs  TsampNgainVariant=Passthrough  TsampIntegralVariant=Disabled_SignalSpec  ExternalSaturationOutDataTypeStr=Inherit: Same as second input  DerivativeSourceVariant=Disabled  PreIntVariant=InternalPreInt
  Vq_ctrl : slpidlib/PID Controller  Controller=PI  Form=Parallel  TimeDomain=Discrete-time  UseExternalTs=off  SampleTime=1/(65e3*10)  IntegratorMethod=Backward Euler  FilterMethod=Forward Euler  ControllerParametersSource=internal  P=-2  I=-.2  UseKiTs=off  D=0  UseExternalDerivativeSource=off  N=100  UseFilter=on  TunerSelectOption=Transfer Function Based (PID Tuner App)  InitialConditionSource=internal  InitialConditionForIntegrator=0  InitialConditionForFilter=0  DifferentiatorICPrevScaledInput=0  ExternalReset=none  TrackingMode=off  Kt=1  LimitOutput=off  SatLimitsSource=internal  UpperSaturationLimit=5e2  LowerSaturationLimit=-5e2  LinearizeAsGain=on  AntiWindupMode=clamping  Kb=1  LimitIntegrator=off  UpperIntegratorSaturationLimit=inf  LowerIntegratorSaturationLimit=-inf  POutMin=[]  POutMax=[]  IOutMin=[]  IOutMax=[]  DOutMin=[]  DOutMax=[]  NOutMin=[]  NOutMax=[]  SumOutMin=[]  SumOutMax=[]  SaturationOutMin=[]  SaturationOutMax=[]  PParamMin=[]  PParamMax=[]  IParamMin=[]  IParamMax=[]  DParamMin=[]  DParamMax=[]  NParamMin=[]  NParamMax=[]  KbParamMin=[]  KbParamMax=[]  KtParamMin=[]  KtParamMax=[]  KbOutMin=[]  KbOutMax=[]  KtOutMin=[]  KtOutMax=[]  IntegratorOutMin=[]  IntegratorOutMax=[]  FilterOutMin=[]  FilterOutMax=[]  SumI1OutMin=[]  SumI1OutMax=[]  SumI2OutMin=[]  SumI2OutMax=[]  SumI3OutMin=[]  SumI3OutMax=[]  SumI4OutMin=[]  SumI4OutMax=[]  SumDOutMin=[]  SumDOutMax=[]  DifferentiatorOutMin=[]  DifferentiatorOutMax=[]  FilterDiffOutCoefMin=[]  FilterDiffOutCoefMax=[]  ReciprocalOutMin=[]  ReciprocalOutMax=[]  SumDenOutMin=[]  SumDenOutMax=[]  SumNumOutMin=[]  SumNumOutMax=[]  DivideOutMin=[]  DivideOutMax=[]  UdiffTsProdOutMin=[]  UdiffTsProdOutMax=[]  NTsProdOutMin=[]  NTsProdOutMax=[]  UintegralTsProdOutMin=[]  UintegralTsProdOutMax=[]  UngainTsProdOutMin=[]  UngainTsProdOutMax=[]  ClampingZeroOutDataTypeStr=Inherit: Inherit via back propagation  ClampingZeroOutMin=[]  ClampingZeroOutMax=[]  FilterDenConstantOutDataTypeStr=Inherit: Inherit via back propagation  FilterDenConstantOutMin=[]  FilterDenConstantOutMax=[]  PCopyOutDataTypeStr=Inherit: Inherit via back propagation  PCopyOutMin=[]  PCopyOutMax=[]  NCopyOutDataTypeStr=Inherit: Inherit via back propagation  NCopyOutMin=[]  NCopyOutMax=[]  IntegratorContinuousStateAttributes=''  IntegratorStateMustResolveToSignalObject=off  IntegratorRTWStateStorageClass=Auto  FilterContinuousStateAttributes=''  FilterStateMustResolveToSignalObject=off  FilterRTWStateStorageClass=Auto  ParallelPVariant=InternalParameters  IdealPVariant=Disabled  IVariant=InternalParameters  DVariant=Disabled  IntegratorVariant=Discrete  SatVariant=Disabled  AWVariant=Passthrough  PCopyVariant=Disabled  TRVariant=Disabled  FdbkBlocksVariant=Forward  IdealPFdbkVariant=Disabled  SatFdbkVariant=Disabled  DerivativeFilterVariant=Disabled  NVariant=Disabled  NCopyVariant=Disabled_SignalSpec  FilterICVariant=Disabled  IntegratorICVariant=InternalICs  ExternalResetVariant=Disabled  TRSumVariant=Passthrough  SumFdbkVariant=Disabled  SumVariant=Sum_PI  TsampFilterVariant=InternalTs  TsampNgainVariant=Passthrough  TsampIntegralVariant=Disabled_SignalSpec  ExternalSaturationOutDataTypeStr=Inherit: Same as second input  DerivativeSourceVariant=Disabled  PreIntVariant=InternalPreInt
  Vd_inductor : Outport
  Vq_inductor : Outport  Port=2
  wires:
  Add3/1 -> Vd_ctrl/1  "error_id"
  id/1 -> Add3/2
  Constant/1 -> Add3/1
  iq/1 -> Add4/2
  Add4/1 -> Vq_ctrl/1  "error_iq"
  Vd_ctrl/1 -> Vd_inductor/1
  Vq_ctrl/1 -> Vq_inductor/1
  Constant1/1 -> Add4/1

== system pfc_desktop_hdl/Subsystem1/ctrl_pwm/SVPWM ==
  Vd_inductor : Inport
  angle : Inport  Port=2
  Vq_inductor : Inport  Port=3
  Cos : Trigonometry  Operator=cos
  Inverse Park Transform : mcbcontrolslib/Inverse Park Transform  PhaseInput=Two inputs  AxisAlignment=D-axis  ThetaInput=Sine and Cosine electrical position  AngleInput=Per-unit  N_points=1024
  SVPWM Generator (2-Level) : spsSVPWMGenerator2LevelLib/SVPWM Generator (2-Level)  InputType=alpha-beta components  SwitchingPattern=Pattern #1  Fc=fsw*1e3  ParUref=[0.8 -30 50]  Ts=t_ss
  Sin : Trigonometry
  P : Outport
  wires:
  Vd_inductor/1 -> Inverse Park Transform/1
  Vq_inductor/1 -> Inverse Park Transform/2
  Inverse Park Transform/2 -> SVPWM Generator (2-Level)/2  "Vbet_indc"
  Sin/1 -> Inverse Park Transform/3
  Cos/1 -> Inverse Park Transform/4
  Inverse Park Transform/1 -> SVPWM Generator (2-Level)/1  "Valp_indc"
  angle/1 -> Cos/1, Sin/1
  SVPWM Generator (2-Level)/1 -> P/1

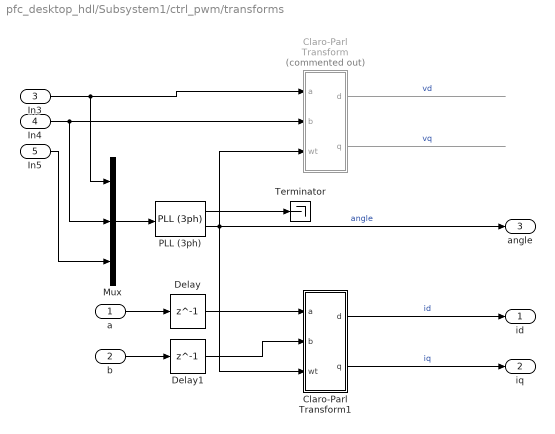
== system pfc_desktop_hdl/Subsystem1/ctrl_pwm/transforms ==
  a : Inport
  b : Inport  Port=2
  In3 : Inport  Port=3
  In4 : Inport  Port=4
  In5 : Inport  Port=5
  Claro-Parl Transform : Subsystem  Commented=on
  Claro-Parl Transform1 : Subsystem
  Delay : Delay  DelayLength=1
  Delay1 : Delay  DelayLength=1
  Mux : Mux  Inputs=3
  PLL (3ph) : spsPLL3phLib/PLL (3ph)  Fmin=50  Par_Init=[0, 50]  ParK=[180,3200,1]  TcD=1e-4  MaxRateChangeFreq=12  FilterCutOffFreq=25  Ts=t_ss  AGC=on
  Terminator : Terminator
  id : Outport
  iq : Outport  Port=2
  angle : Outport  Port=3
  wires:
  Mux/1 -> PLL (3ph)/1
  PLL (3ph)/2 -> angle/1, Claro-Parl Transform1/3(wt), Claro-Parl Transform/3(wt)  "angle"
  PLL (3ph)/1 -> Terminator/1
  In3/1 -> Mux/1, Claro-Parl Transform/1(a)
  In5/1 -> Mux/3
  b/1 -> Delay1/1
  In4/1 -> Claro-Parl Transform/2(b), Mux/2
  a/1 -> Delay/1
  Delay/1 -> Claro-Parl Transform1/1(a)
  Delay1/1 -> Claro-Parl Transform1/2(b)
  Claro-Parl Transform/1(d) -> ?  "vd"
  Claro-Parl Transform/2(q) -> ?  "vq"
  Claro-Parl Transform1/1(d) -> id/1  "id"
  Claro-Parl Transform1/2(q) -> iq/1  "iq"

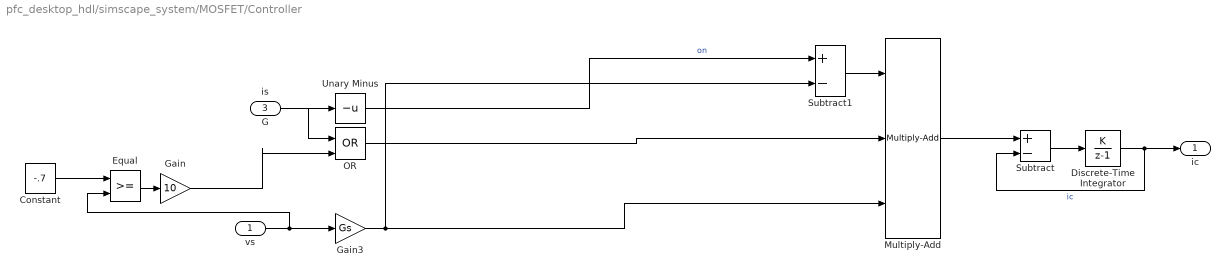
== system pfc_desktop_hdl/simscape_system/MOSFET/Controller ==
  vs : Inport
  is : Inport  Port=2
  G : Inport  Port=3
  Constant : Constant  Value=-.7  SampleTime=-1
  Discrete-Time Integrator : DiscreteIntegrator  IntegratorMethod=Accumulation: Forward Euler  gainval=1/s  SampleTime=-1  OutDataTypeStr=Inherit: Inherit via back propagation  ICPrevOutput=DiscIntNeverNeededParam  ICPrevScaledInput=DiscIntNeverNeededParam
  Equal : RelationalOperator  OutDataTypeStr=boolean  RndMeth=Simplest  InputSameDT=off
  Gain : Gain  Gain=10
  Gain3 : Gain  Gain=Gs  OutDataTypeStr=Inherit: Inherit via back propagation
  Multiply-Add : hdlsllib/HDL Operations/Multiply-Add  Function=c+(a.*b)  datatype=Inherit: Inherit via internal rule  DoSatur=off  FMA=off
      settings: LibrarySourceBlock=SimscapeFPGAHIL_lib/Linearized Switch Models/Switch/Controller/Switch State/Subcycle Average (Floating-Point)/Multiply-Add
  OR : Logic  Operator=OR  IconShape=distinctive  AllPortsSameDT=off  OutDataTypeStr=boolean
  Subtract : Sum  Inputs=+-
  Subtract1 : Sum  Inputs=+-
  Unary Minus : UnaryMinus
  ic : Outport
  wires:
  Multiply-Add/1 -> Subtract/1
  G/1 -> OR/1
  Unary Minus/1 -> Subtract1/1  "on"
  is/1 -> Unary Minus/1
  Discrete-Time Integrator/1 -> ic/1, Subtract/2  "ic"
  Subtract/1 -> Discrete-Time Integrator/1
  vs/1 -> Equal/2, Gain3/1
  Equal/1 -> Gain/1
  Gain/1 -> OR/2
  Constant/1 -> Equal/1
  Gain3/1 -> Subtract1/2, Multiply-Add/3
  Subtract1/1 -> Multiply-Add/1
  OR/1 -> Multiply-Add/2

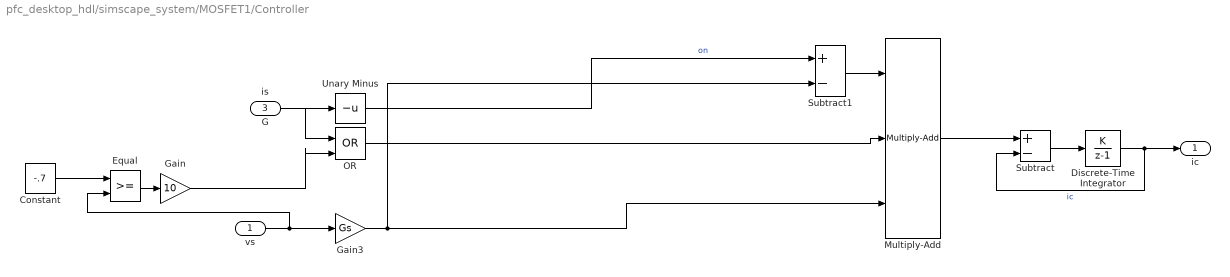
== system pfc_desktop_hdl/simscape_system/MOSFET1/Controller ==
  vs : Inport
  is : Inport  Port=2
  G : Inport  Port=3
  Constant : Constant  Value=-.7  SampleTime=-1
  Discrete-Time Integrator : DiscreteIntegrator  IntegratorMethod=Accumulation: Forward Euler  gainval=1/s  SampleTime=-1  OutDataTypeStr=Inherit: Inherit via back propagation  ICPrevOutput=DiscIntNeverNeededParam  ICPrevScaledInput=DiscIntNeverNeededParam
  Equal : RelationalOperator  OutDataTypeStr=boolean  RndMeth=Simplest  InputSameDT=off
  Gain : Gain  Gain=10
  Gain3 : Gain  Gain=Gs  OutDataTypeStr=Inherit: Inherit via back propagation
  Multiply-Add : hdlsllib/HDL Operations/Multiply-Add  Function=c+(a.*b)  datatype=Inherit: Inherit via internal rule  DoSatur=off  FMA=off
  OR : Logic  Operator=OR  IconShape=distinctive  AllPortsSameDT=off  OutDataTypeStr=boolean
  Subtract : Sum  Inputs=+-
  Subtract1 : Sum  Inputs=+-
  Unary Minus : UnaryMinus
  ic : Outport
  wires:
  OR/1 -> Multiply-Add/2
  Subtract1/1 -> Multiply-Add/1
  Gain3/1 -> Multiply-Add/3, Subtract1/2
  Constant/1 -> Equal/1
  Gain/1 -> OR/2
  Equal/1 -> Gain/1
  vs/1 -> Gain3/1, Equal/2
  Subtract/1 -> Discrete-Time Integrator/1
  Discrete-Time Integrator/1 -> Subtract/2, ic/1  "ic"
  is/1 -> Unary Minus/1
  Unary Minus/1 -> Subtract1/1  "on"
  G/1 -> OR/1
  Multiply-Add/1 -> Subtract/1

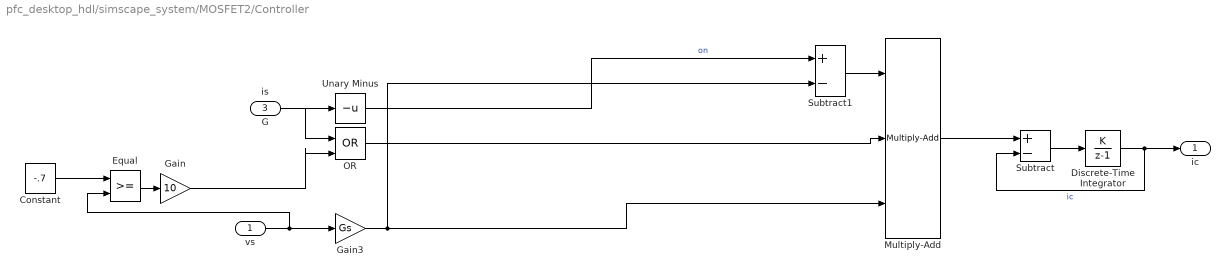
== system pfc_desktop_hdl/simscape_system/MOSFET2/Controller ==
  vs : Inport
  is : Inport  Port=2
  G : Inport  Port=3
  Constant : Constant  Value=-.7  SampleTime=-1
  Discrete-Time Integrator : DiscreteIntegrator  IntegratorMethod=Accumulation: Forward Euler  gainval=1/s  SampleTime=-1  OutDataTypeStr=Inherit: Inherit via back propagation  ICPrevOutput=DiscIntNeverNeededParam  ICPrevScaledInput=DiscIntNeverNeededParam
  Equal : RelationalOperator  OutDataTypeStr=boolean  RndMeth=Simplest  InputSameDT=off
  Gain : Gain  Gain=10
  Gain3 : Gain  Gain=Gs  OutDataTypeStr=Inherit: Inherit via back propagation
  Multiply-Add : hdlsllib/HDL Operations/Multiply-Add  Function=c+(a.*b)  datatype=Inherit: Inherit via internal rule  DoSatur=off  FMA=off
  OR : Logic  Operator=OR  IconShape=distinctive  AllPortsSameDT=off  OutDataTypeStr=boolean
  Subtract : Sum  Inputs=+-
  Subtract1 : Sum  Inputs=+-
  Unary Minus : UnaryMinus
  ic : Outport
  wires:
  Multiply-Add/1 -> Subtract/1
  G/1 -> OR/1
  Unary Minus/1 -> Subtract1/1  "on"
  is/1 -> Unary Minus/1
  Discrete-Time Integrator/1 -> ic/1, Subtract/2  "ic"
  Subtract/1 -> Discrete-Time Integrator/1
  vs/1 -> Equal/2, Gain3/1
  Equal/1 -> Gain/1
  Gain/1 -> OR/2
  Constant/1 -> Equal/1
  Gain3/1 -> Subtract1/2, Multiply-Add/3
  Subtract1/1 -> Multiply-Add/1
  OR/1 -> Multiply-Add/2

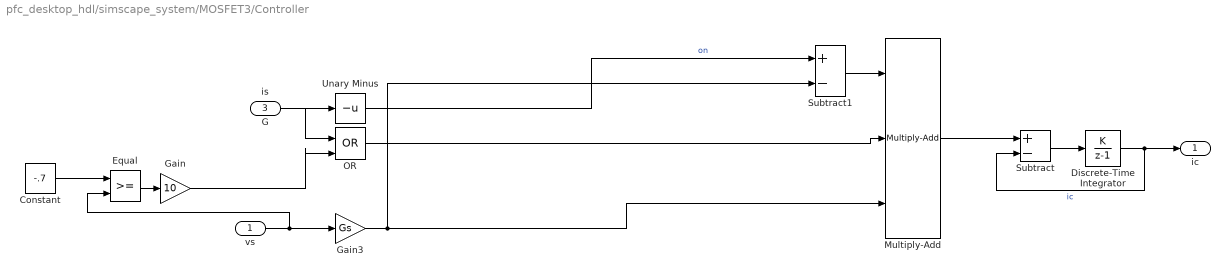
== system pfc_desktop_hdl/simscape_system/MOSFET3/Controller ==
  vs : Inport
  is : Inport  Port=2
  G : Inport  Port=3
  Constant : Constant  Value=-.7  SampleTime=-1
  Discrete-Time Integrator : DiscreteIntegrator  IntegratorMethod=Accumulation: Forward Euler  gainval=1/s  SampleTime=-1  OutDataTypeStr=Inherit: Inherit via back propagation  ICPrevOutput=DiscIntNeverNeededParam  ICPrevScaledInput=DiscIntNeverNeededParam
  Equal : RelationalOperator  OutDataTypeStr=boolean  RndMeth=Simplest  InputSameDT=off
  Gain : Gain  Gain=10
  Gain3 : Gain  Gain=Gs  OutDataTypeStr=Inherit: Inherit via back propagation
  Multiply-Add : hdlsllib/HDL Operations/Multiply-Add  Function=c+(a.*b)  datatype=Inherit: Inherit via internal rule  DoSatur=off  FMA=off
  OR : Logic  Operator=OR  IconShape=distinctive  AllPortsSameDT=off  OutDataTypeStr=boolean
  Subtract : Sum  Inputs=+-
  Subtract1 : Sum  Inputs=+-
  Unary Minus : UnaryMinus
  ic : Outport
  wires:
  OR/1 -> Multiply-Add/2
  Subtract1/1 -> Multiply-Add/1
  Gain3/1 -> Multiply-Add/3, Subtract1/2
  Constant/1 -> Equal/1
  Gain/1 -> OR/2
  Equal/1 -> Gain/1
  vs/1 -> Gain3/1, Equal/2
  Subtract/1 -> Discrete-Time Integrator/1
  Discrete-Time Integrator/1 -> Subtract/2, ic/1  "ic"
  is/1 -> Unary Minus/1
  Unary Minus/1 -> Subtract1/1  "on"
  G/1 -> OR/1
  Multiply-Add/1 -> Subtract/1
